simulink model "nonlinear_model"  (R2016a)
settings: Solver=VariableStepAuto  StartTime=0.0  StopTime=2.28  RelTol=1e-3
settings Model: Creator=kreitzem  LastModifiedBy=kreitzem

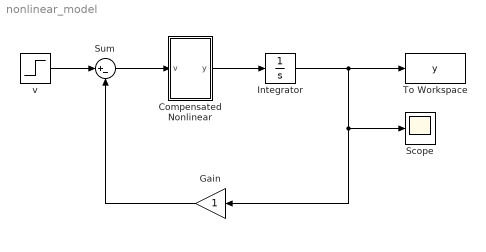
== system nonlinear_model ==
  "Compensated Nonlinear " : Subsystem
  Gain : Gain
  Integrator : Integrator
  Scope : Scope
  Sum : Sum  Inputs=|+-
  To Workspace : ToWorkspace  VariableName=y  SaveFormat=Timeseries  SampleTime=-1
  v : Step  SampleTime=0
  wires:
  v/1 -> Sum/1
  Gain/1 -> Sum/2
  "Compensated Nonlinear "/1(y) -> Integrator/1
  Sum/1 -> "Compensated Nonlinear "/1(v)
  Integrator/1 -> Gain/1, Scope/1, To Workspace/1

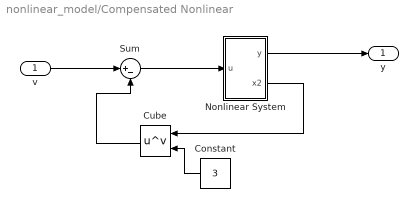
== system nonlinear_model/Compensated Nonlinear  ==
  v : Inport
  Constant : Constant  Value=3
  Cube : Math  Operator=pow  SaturateOnIntegerOverflow=on
  Nonlinear System : Subsystem
  Sum : Sum  Inputs=|+-
  y : Outport
  wires:
  Nonlinear System/1(y) -> y/1
  Nonlinear System/2(x2) -> Cube/1
  Cube/1 -> Sum/2
  Constant/1 -> Cube/2
  Sum/1 -> Nonlinear System/1(u)
  v/1 -> Sum/1

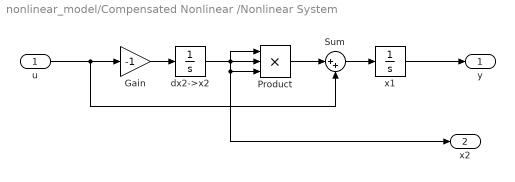
== system nonlinear_model/Compensated Nonlinear /Nonlinear System ==
  u : Inport
  Gain : Gain  Gain=-1
  Product : Product  Inputs=3
  Sum : Sum  Inputs=|++
  "dx2->x2 " : Integrator  InitialCondition=1e-12
  x1 : Integrator  InitialCondition=1e-12
  y : Outport
  x2 : Outport  Port=2
  wires:
  x1/1 -> y/1
  "dx2->x2 "/1 -> x2/1, Product/3, Product/2, Product/1
  Product/1 -> Sum/1
  Gain/1 -> "dx2->x2 "/1
  u/1 -> Gain/1, Sum/2
  Sum/1 -> x1/1
